simulink model "observer1"  (Simulink 7.7)
settings: Solver=ode45  StartTime=0.0  StopTime=10  RelTol=1e-3
values from neighbouring files (symbols this model uses):
  A = load('HW4_Amatrix.dat')    [script1.m]    (also in script2.m; script3.m)
  B = load('HW4_Bmatrix.dat')    [script1.m]    (also in script2.m; script3.m)
  C = load('HW4_Cmatrix.dat')    [script1.m]    (also in script2.m = eye(9); script3.m)
  D = load('HW4_Dmatrix.dat')    [script1.m]    (also in script2.m = zeros(9,3); script3.m = zeros(9,3))
  k = lqr(A,B,Q,R)    [script1.m]    (also in script2.m = LQR(A,B,Q,R); script3.m = LQR(A,B,Q,R))
  L = lqr(A',C',Q1,R1)    [script1.m]
  x0 = [0 0 0 0 0 0 0 0 0]'    [script1.m]    (also in script2.m; script3.m)
settings Model: Creator=Dell  LastModifiedBy=Dell
settings DataIOCC: LimitDataPoints=off

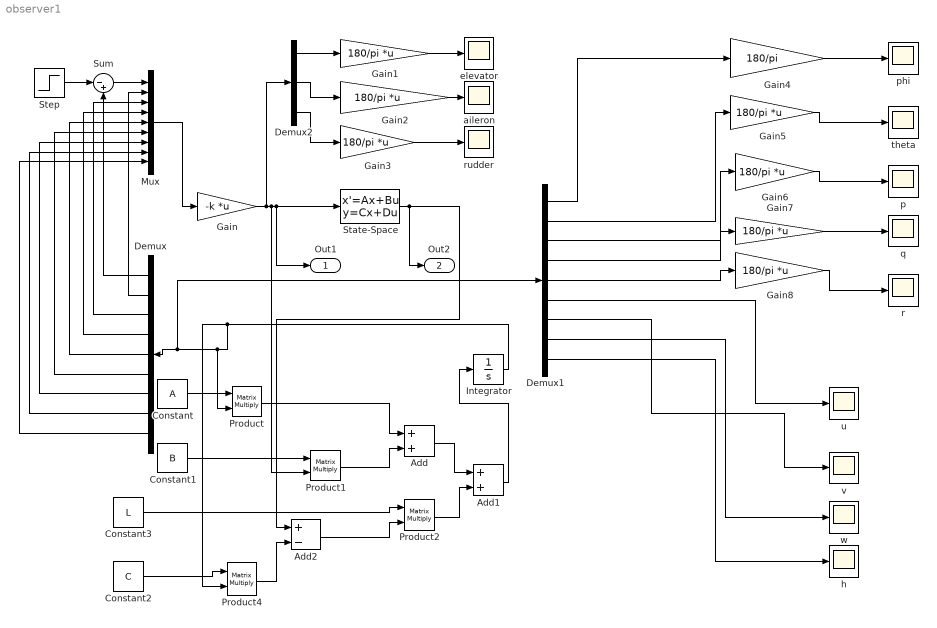
== system observer1 ==
  Add : Sum
  Add1 : Sum
  Add2 : Sum  Inputs=+-
  Constant : Constant  Value=A
  Constant1 : Constant  Value=B
  Constant2 : Constant  Value=C
  Constant3 : Constant  Value=L
  Demux : Demux  Outputs=9
  Demux1 : Demux  Outputs=9
  Demux2 : Demux  Outputs=3
  Gain : Gain  Gain=-k  Multiplication=Matrix(K*u)
  Gain{1..3,5..8} (7 alike) : Gain  Gain=180/pi  Multiplication=Matrix(K*u)
  Gain4 : Gain  Gain=180/pi
  Integrator : Integrator
  Mux : Mux  Inputs=9
  Product{,1..2,4} (4 alike) : Product  Multiplication=Matrix(*)  RndMeth=Zero
  State-Space : StateSpace  A=A  B=B  C=C  D=D  X0=x0
  Step : Step  Time=1*pi/180  After=30*pi/180  SampleTime=0
  Sum : Sum  Inputs=|-+
  aileron : Scope
      settings: SaveName=ScopeData2
  elevator : Scope
  h : Scope
  p : Scope
      settings: SaveName=ScopeData6
  phi : Scope
      settings: SaveName=ScopeData4
  q : Scope
      settings: SaveName=ScopeData7
  r : Scope
      settings: SaveName=ScopeData8
  rudder : Scope
      settings: SaveName=ScopeData3
  theta : Scope
      settings: SaveName=ScopeData5
  u : Scope
      settings: SaveName=ScopeData9
  v : Scope
      settings: SaveName=ScopeData10
  w : Scope
      settings: SaveName=ScopeData11
  Out1 : Outport
  Out2 : Outport  Port=2
  wires:
  Step/1 -> Sum/1
  Sum/1 -> Mux/1
  Demux/1 -> Sum/2
  Demux/2 -> Mux/2
  Demux/3 -> Mux/3
  Demux/4 -> Mux/4
  Demux/5 -> Mux/5
  Demux/6 -> Mux/6
  Demux/7 -> Mux/7
  Demux/8 -> Mux/8
  Demux/9 -> Mux/9
  Mux/1 -> Gain/1
  Gain/1 -> Demux2/1, Out1/1, State-Space/1, Product1/2
  Demux2/1 -> Gain1/1
  Demux2/2 -> Gain2/1
  Demux2/3 -> Gain3/1
  Gain1/1 -> elevator/1
  State-Space/1 -> Out2/1, Add2/1
  Demux1/1 -> Gain4/1
  Demux1/2 -> Gain5/1
  Demux1/3 -> Gain6/1
  Demux1/4 -> Gain7/1
  Demux1/5 -> Gain8/1
  Demux1/6 -> u/1
  Demux1/7 -> v/1
  Demux1/8 -> w/1
  Demux1/9 -> h/1
  Gain4/1 -> phi/1
  Gain5/1 -> theta/1
  Gain6/1 -> p/1
  Gain7/1 -> q/1
  Gain8/1 -> r/1
  Gain2/1 -> aileron/1
  Gain3/1 -> rudder/1
  Product/1 -> Add/1
  Product1/1 -> Add/2
  Product2/1 -> Add1/2
  Add/1 -> Add1/1
  Add1/1 -> Integrator/1
  Integrator/1 -> Product4/2, Product/2, Demux1/1, Demux/1
  Constant1/1 -> Product1/1
  Constant2/1 -> Product4/1
  Product4/1 -> Add2/2
  Constant3/1 -> Product2/1
  Add2/1 -> Product2/2
  Constant/1 -> Product/1
